simulink model "EV_Powertrain_Simulation"  (R2025b)
settings: Solver=VariableStepAuto  StartTime=0.0  StopTime=10.0  RelTol=1e-3
libraries: simulink x1
settings Model: Creator=gaura  LastModifiedBy=gaura

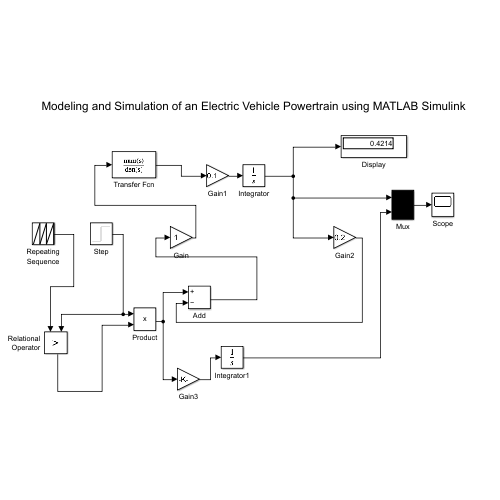
[thumbnail: Simulink's stored preview of the top-level diagram]
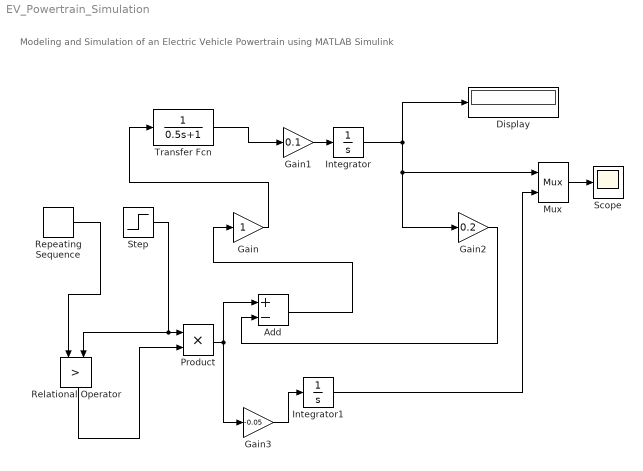
== system EV_Powertrain_Simulation ==
  note: Modeling and Simulation of an Electric Vehicle Powertrain using MATLAB Simulink
  Add : Sum  Inputs=+-
  Display : Display
  Gain : Gain
  Gain1 : Gain  Gain=0.1
  Gain2 : Gain  Gain=0.2
  Gain3 : Gain  Gain=-0.05
  Integrator : Integrator
  Integrator1 : Integrator  InitialCondition=1
  Mux : Mux  Inputs=2
  Product : Product
  Relational Operator : RelationalOperator  Operator=>  OutDataTypeStr=boolean  RndMeth=Simplest  InputSameDT=off
  Repeating Sequence : simulink/Sources/Repeating Sequence  rep_seq_t=[0 2]  rep_seq_y=[0 2]
  Scope : Scope
      settings: ActiveDisplayYMinimum=-1.8200818298619903  ActiveDisplayYMaximum=5.40158891181715
  Step : Step  SampleTime=0
  Transfer Fcn : TransferFcn  Denominator=[0.5 1]
  wires:
  Transfer Fcn/1 -> Gain1/1
  Gain2/1 -> Add/2
  Add/1 -> Gain/1
  Integrator/1 -> Gain2/1, Mux/1, Display/1
  Gain/1 -> Transfer Fcn/1
  Gain1/1 -> Integrator/1
  Step/1 -> Product/1, Relational Operator/2
  Relational Operator/1 -> Product/2
  Product/1 -> Gain3/1, Add/1
  Repeating Sequence/1 -> Relational Operator/1
  Gain3/1 -> Integrator1/1
  Mux/1 -> Scope/1
  Integrator1/1 -> Mux/2
